simulink model "MPC_Speed_Control"  (R2024b)
settings: Solver=VariableStepAuto  StartTime=0.0  StopTime=50  RelTol=1e-3
model workspace (MAT data in the model file):
  I_max = Simulink.Parameter
  I_max.Complexity = 'real'
  I_max.Dimensions = [0 0]
  I_max.DataType = 'auto'
  Iq_max = Simulink.Parameter
  Iq_max.Value = 20
  Iq_max.Complexity = 'real'
  Iq_max.Dimensions = [1 1]
  Iq_max.DataType = 'double'
  Iq_max.Min = 0
  Iq_max.Max = 20
  Iq_max.DocUnits = 'A'
  Mech_Load = Simulink.Parameter
  Mech_Load.Value = 1
  Mech_Load.Complexity = 'real'
  Mech_Load.Dimensions = [1 1]
  Mech_Load.DataType = 'double'
  Mech_Load.Min = 0
  Mech_Load.Max = 20
libraries: spsCurrentMeasurementLib x3, spsSeriesRLCBranchLib x3, spsVoltageMeasurementLib x2, spsDCVoltageSourceLib x1, spsGroundLib x1, spsPermanentMagnetSynchronousMachineLib x1, spsUniversalBridgeLib x1, spsRMSLib x1, eeTransforms x1, slpidlib x1, spspowerguiLib x1
settings Model: ParameterArgumentNames=Iq_max,Mech_Load  Creator=hp  LastModifiedBy=hp
settings RTWCC: RTWVerbose=off

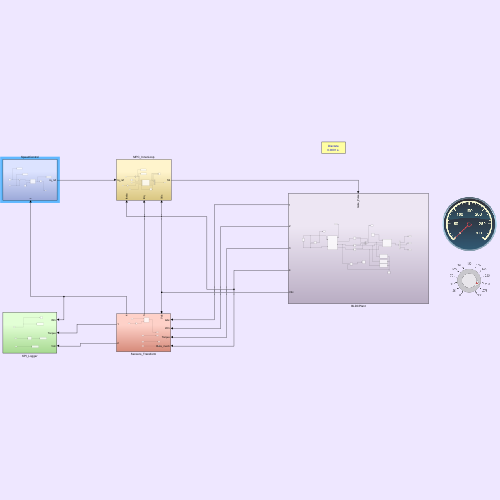
[thumbnail: Simulink's stored preview of the top-level diagram]
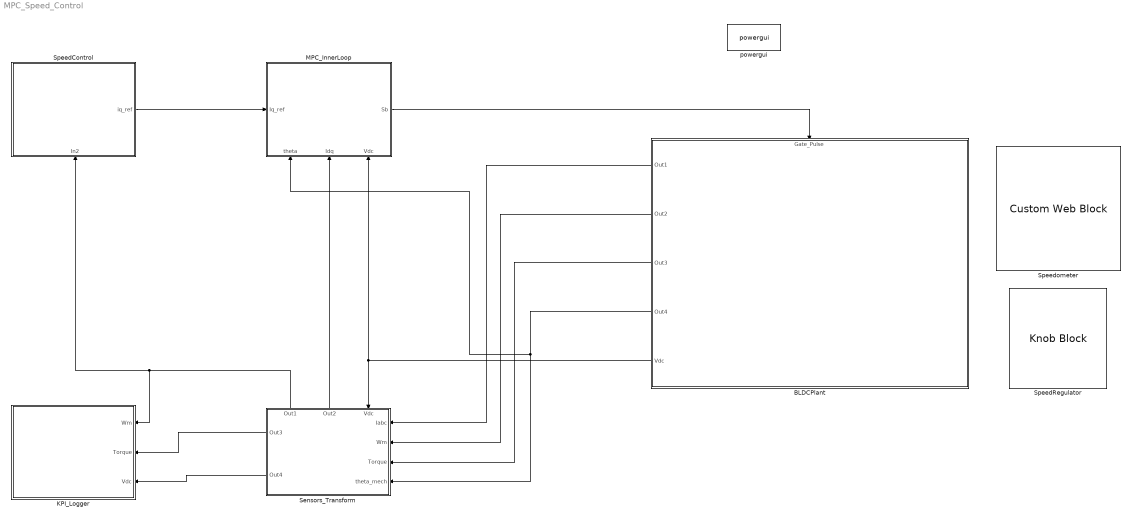
== system MPC_Speed_Control ==
  BLDCPlant : Subsystem
      settings: PortSchema="{\"entries\":[{\"content\":{\"sides\":[{\"content\":{},\"type\":\"ConnectorPlacement.EquallySpacedRectSide\",\"uuid\":\"b62d1c6e-a59d-4f65-8814-3dc177b23cd5\"},{\"content\":{\"connectorIds\":[\"Out1\",\"Out2\",\"Out3\",\"Out4\",\"Out5\"],\"side\":\"RIGHT\"},\"type\":\"ConnectorPlacement.EquallySpacedRectSide\",\"uuid\":\"6a33075d-b69e-43e0-847d-75198eb85e92\"},{\"content\":{\"connectorIds\":[\"In1\"],\"side\":\"TOP\"},\"type\":\"ConnectorPlacement.EquallySpacedRectSide\",\"uuid\":\"25902762-9f38-46cd-ae2e-4756f044da85\"}]},\"type\":\"ConnectorPlacement.EquallySpacedConnector\",\"uuid\":\"f42ce1bc-9199-4fe0-a1c0-02ea16a986e3\"}],\"packageUris\":[\"http://schema.mathworks.com/mf0/Connector/R2020b\"],\"version\":\"1.0\"}"
  KPI_Logger : Subsystem
  MPC_InnerLoop : Subsystem
      settings: PortSchema="{\"entries\":[{\"content\":{\"sides\":[{\"content\":{\"connectorIds\":[\"In1\"]},\"type\":\"ConnectorPlacement.EquallySpacedRectSide\",\"uuid\":\"1cededfe-a157-4693-a5d6-3ded835fc0fc\"},{\"content\":{\"connectorIds\":[\"Out1\"],\"side\":\"RIGHT\"},\"type\":\"ConnectorPlacement.EquallySpacedRectSide\",\"uuid\":\"33a5264e-419d-490c-8c5a-eb4ad8051faa\"},{\"content\":{\"side\":\"TOP\"},\"type\":\"ConnectorPlacement.EquallySpacedRectSide\",\"uuid\":\"1a0bf29c-4856-430c-b6c2-7eb59e496e99\"},{\"content\":{\"connectorIds\":[\"In2\",\"In3\",\"In4\"],\"side\":\"BOTTOM\"},\"type\":\"ConnectorPlacement.EquallySpacedRectSide\",\"uuid\":\"91ee846a-69f5-4705-a04e-f801c9f974eb\"}]},\"type\":\"ConnectorPlacement.EquallySpacedConnector\",\"uuid\":\"2fb1adc4-a0ec-4398-a1b1-d31f9fed8fac\"}],\"packageUris\":[\"http://schema.mathworks.com/mf0/Connector/R2020b\"],\"version\":\"1.0\"}"
  Sensors_Transform : Subsystem
      settings: PortSchema="{\"entries\":[{\"content\":{\"sides\":[{\"content\":{\"connectorIds\":[\"In1\",\"In2\",\"In3\",\"In4\"]},\"type\":\"ConnectorPlacement.EquallySpacedRectSide\",\"uuid\":\"6e3abafc-9605-4c64-93b2-a4bb92d8b15c\"},{\"content\":{\"connectorIds\":[\"Out1\",\"Out2\"],\"side\":\"RIGHT\"},\"type\":\"ConnectorPlacement.EquallySpacedRectSide\",\"uuid\":\"b2aa59f5-86cc-4d40-acb7-825075212f50\"},{\"content\":{\"connectorIds\":[\"In5\",\"Out3\",\"Out4\"],\"side\":\"TOP\"},\"type\":\"ConnectorPlacement.EquallySpacedRectSide\",\"uuid\":\"761892ed-2e7f-4fbb-8f28-8445ea92004b\"},{\"content\":{\"side\":\"BOTTOM\"},\"type\":\"ConnectorPlacement.EquallySpacedRectSide\",\"uuid\":\"9c48b8cc-eb13-4556-8d10-7bc854d50a3a\"}]},\"type\":\"ConnectorPlacement.EquallySpacedConnector\",\"uuid\":\"5da58205-14da-4f32-a3a9-21dbad898aea\"}],\"packageUris\":[\"http://schema.mathworks.com/mf0/Connector/R2020b\"],\"version\":\"1.0\"}"
  SpeedControl : Subsystem
      settings: PortSchema="{\"entries\":[{\"content\":{\"sides\":[{\"content\":{},\"type\":\"ConnectorPlacement.EquallySpacedRectSide\",\"uuid\":\"1cededfe-a157-4693-a5d6-3ded835fc0fc\"},{\"content\":{\"connectorIds\":[\"Out1\"],\"side\":\"RIGHT\"},\"type\":\"ConnectorPlacement.EquallySpacedRectSide\",\"uuid\":\"33a5264e-419d-490c-8c5a-eb4ad8051faa\"},{\"content\":{\"side\":\"TOP\"},\"type\":\"ConnectorPlacement.EquallySpacedRectSide\",\"uuid\":\"1a0bf29c-4856-430c-b6c2-7eb59e496e99\"},{\"content\":{\"connectorIds\":[\"In1\"],\"side\":\"BOTTOM\"},\"type\":\"ConnectorPlacement.EquallySpacedRectSide\",\"uuid\":\"33f77dac-6bdc-4222-b29b-be44d81ff2fe\"}]},\"type\":\"ConnectorPlacement.EquallySpacedConnector\",\"uuid\":\"2fb1adc4-a0ec-4398-a1b1-d31f9fed8fac\"}],\"packageUris\":[\"http://schema.mathworks.com/mf0/Connector/R2020b\"],\"version\":\"1.0\"}"
  SpeedRegulator : KnobBlock  LabelPosition=Hide  ScaleMax=300
  Speedometer : CustomWebBlock  LabelPosition=Hide  ShowInitialText=on  Configuration="{\"components\":[{\"name\":\"CircularScaleComponent\",\"settings\":{\"bounds\":{\"max\":300,\"min\":0,\"tickInterval\":\"auto\"},\"direction\":\"cw\",\"flipLimits\":0,\"innerRadius\":0.75,\"internalTickHeightScaleFactor\":1,\"labelColor\":[255,255,200],\"labelFont\":{\"font\":\"Arial\",\"fontSize\":12},\"labelRadius\":0.528,\"labelTransparency\":1,\"minorTickHeightScaleFactor\":0.2,\"needleImage\":{\"size\":[200,50],\"src\":\"data:image\\/svg+xml;base64,PD94bWwgdmVyc2lvbj0iMS4wIiBlbmNvZGluZz0idXRmLTgiPz4KPCEtLSBHZW5lcmF0b3I6IEFkb2JlIElsbHVzdHJhdG9yIDI0LjEuMiwgU1ZHIEV4cG9ydCBQbHVnLUluIC4gU1ZHIFZlcnNpb246IDYuMDAgQnVpbGQgMCkgIC0tPgo8c3ZnIHZlcnNpb249IjEuMSIgaWQ9IkxheWVyXzEiIHhtbG5zPSJodHRwOi8vd3d3LnczLm9yZy8yMDAwL3N2ZyIgeG1sbnM6eGxpbms9Imh0dHA6Ly93d3cudzMub3JnLzE5OTkveGxpbmsiIHg9IjBweCIgeT0iMHB4IgoJIHZpZXdCb3g9IjAgMCAyMDAgNTAiIHN0eWxlPSJlbmFibGUtYmFja2dyb3VuZDpuZXcgMCAwIDIwMCA1MDsiIHhtbDpzcGFjZT0icHJlc2VydmUiPgo8c3R5bGUgdHlwZT0idGV4dC9jc3MiPgoJLnN0MHtmaWxsOiNFQzIxMjc7fQo8L3N0eWxlPgo8cGF0aCBjbGFzcz0ic3QwIiBkPSJNMTYyLjgsMTMuN0MxNjksNC40LDE4MS43LDEuOSwxOTEsOC4xczExLjgsMTguOSw1LjYsMjguMnMtMTguOSwxMS44LTI4LjIsNS42bDAsMAoJQzE1OS4xLDM1LjYsMTU2LjYsMjMsMTYyLjgsMTMuN0wxNjIuOCwxMy43eiBNMTY1LjgsMTUuOGMtNS4xLDcuNi0zLjEsMTcuOSw0LjYsMjNjNy42LDUuMSwxNy45LDMuMSwyMy00LjYKCWM1LjEtNy42LDMuMS0xNy45LTQuNi0yM2wwLDBDMTgxLjIsNi4yLDE3MC45LDguMiwxNjUuOCwxNS44eiIvPgo8cGF0aCBjbGFzcz0ic3QwIiBkPSJNMC40LDI1Ljl2LTMuM2wxNTktMi41Yy0wLjcsMi42LTAuNyw1LjIsMCw3LjhMMC40LDI1Ljl6Ii8+CjxjaXJjbGUgY2xhc3M9InN0MCIgY3g9IjE3OS42IiBjeT0iMjQiIHI9IjAuNyIvPgo8L3N2Zz4K\"},\"needleOffset\":[0.18464878250906522,0],\"needleOrientation\":-45,\"needleRotation\":180,\"needleSize\":{\"height\":0.11741692305346914,\"width\":0.46108337545091255},\"outerRadius\":0.9,\"position\":[0.05,0.05,0.9,0.9],\"referencePoint\":\"auto\",\"scaleAngle\":270,\"scaleAngleOffset\":135,\"scaleColors\":[],\"scaleColorsSize\":0.2,\"scaleDirection\":\"CW\",\"scalePosition\":[0,0,1,1],\"showLabels\":1,\"showMinorTicks\":1,\"showSpanLine\":1,\"showTicks\":1,\"tickColor\":[252,252,197],\"tickTransparency\":1,\"valueBarColor\":[0,114,189],\"valueBarPosition\":[0,0,1,1],\"valueBarSize\":0.2,\"valueBarTransparency\":1}},{\"name\":\"BackgroundImageComponent\",\"settings\":{\"image\":{\"size\":[500,500],\"src\":\"data:image\\/svg+xml;base64,PD94bWwgdmVyc2lvbj0iMS4wIiBlbmNvZGluZz0iVVRGLTgiIHN0YW5kYWxvbmU9Im5vIj8+CjxzdmcKICAgeG1sbnM6ZGM9Imh0dHA6Ly9wdXJsLm9yZy9kYy9lbGVtZW50cy8xLjEvIgogICB4bWxuczpjYz0iaHR0cDovL2NyZWF0aXZlY29tbW9ucy5vcmcvbnMjIgogICB4bWxuczpyZGY9Imh0dHA6Ly93d3cudzMub3JnLzE5OTkvMDIvMjItcmRmLXN5bnRheC1ucyMiCiAgIHhtbG5zOnN2Zz0iaHR0cDovL3d3dy53My5vcmcvMjAwMC9zdmciCiAgIHhtbG5zPSJodHRwOi8vd3d3LnczLm9yZy8yMDAwL3N2ZyIKICAgeG1sbnM6 ...(+9964 chars)\"},\"position\":[0,0,1,1],\"scaleMode\":\"0\"}},{\"name\":\"ForegroundImageComponent\",\"settings\":{\"image\":{\"size\":[0,0],\"src\":\"default\",\"srcOrientation\":[]},\"isForeground\":1,\"position\":[0,0,1,1],\"scaleMode\":\"0\"}}],\"settings\":{\"BindingType\":\"signal\",\"aspectRatio\":1.032258064516129,\"backgroundColor\":[0,0,0,\"1\"],\"backgroundOffset\":1,\"backgroundOpacity\":1,\"direction\":\"cw\",\"fixedAspectRatio\":\"on\",\"flipLimits\":0,\"orientation\":\"horizontal\",\"showBackgroundColor\":false,\"value\":0,\"version\":\"R2023a\"},\"type\":\"CircularGauge\"}"
  powergui : spspowerguiLib/powergui  Priority=1  SimulationMode=Discrete  SampleTime=100*1e-6  frequency=60  Iterations=50  frequencyindice=0  Pbase=100e6  ErrMax=1e-4  UnitsV=kV  UnitsW=MW  buscounter=0  FunctionMessages=off  echomessages=off  EnableUseOfTLC=off  CurrentSourceSwitches=off  DisableSnubberDevices=off  DisableRonSwitches=off  DisableVfSwitches=off  DisplayEquations=off  AutomaticDiscreteSolvers=off  SolverType=Tustin/Backward Euler (TBE)  Interpol=off  ExternalGateDelay=off  methode=off  Ts=100  x0status=blocks  SPID=on  SwTol=0  HookPort=off  NonlinearTolerance=1e-4  nMaxIteration=100  ContinueOnMaxIteration=off  RestoreLinks=warning  ResistiveCurrentMeasurement=off  Frange=[0:2:500]  Ylog=off  Xlog=on  ShowGrid=off  save=off  variable=ZData  structure=0  ZoomFFT=off  StartTime=0.0  cycles=1  DisplayStyle=1  fundamental=60  FreqAxis=off  MaxFrequency=1000  frequencyindicesteady=1  RmsSteady=1  display=off
  wires:
  SpeedControl/1(iq_ref) -> MPC_InnerLoop/1(Iq_ref)
  MPC_InnerLoop/1(Sb) -> BLDCPlant/1(Gate_Pulse)
  BLDCPlant/1(Out1) -> Sensors_Transform/1(Iabc)
  Sensors_Transform/4(Out1) -> SpeedControl/1(In2), KPI_Logger/1(Wm)
  Sensors_Transform/3(Out2) -> MPC_InnerLoop/3(Idq)
  Sensors_Transform/1(Out3) -> KPI_Logger/2(Torque)
  BLDCPlant/3(Out3) -> Sensors_Transform/3(Torque)
  BLDCPlant/4(Out4) -> MPC_InnerLoop/2(theta), Sensors_Transform/4(theta_mech)
  BLDCPlant/2(Out2) -> Sensors_Transform/2(Wm)
  BLDCPlant/5(Vdc) -> Sensors_Transform/5(Vdc), MPC_InnerLoop/4(Vdc)
  Sensors_Transform/2(Out4) -> KPI_Logger/3(Vdc)

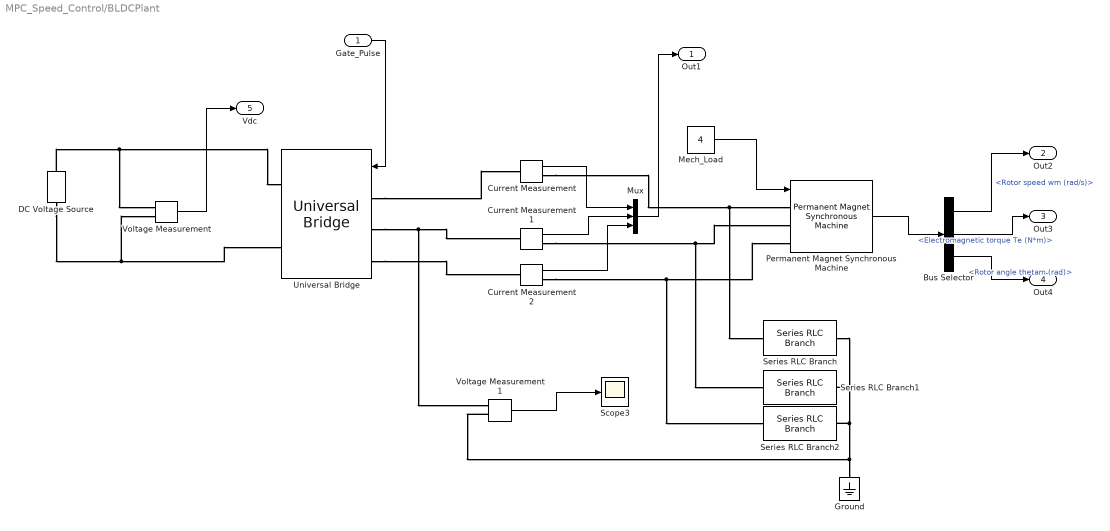
== system MPC_Speed_Control/BLDCPlant ==
  Gate_Pulse : Inport
  Bus Selector : BusSelector  OutputSignals=Rotor speed wm (rad/s),Electromagnetic torque Te (N*m),Rotor angle thetam (rad)
  Current Measurement : spsCurrentMeasurementLib/Current Measurement  PhasorSimulation=off  OutputType=Complex  PSBequivalent=0
  Current Measurement1 : spsCurrentMeasurementLib/Current Measurement  PhasorSimulation=off  OutputType=Complex  PSBequivalent=0
  Current Measurement2 : spsCurrentMeasurementLib/Current Measurement  PhasorSimulation=off  OutputType=Complex  PSBequivalent=0
  DC Voltage Source : spsDCVoltageSourceLib/DC Voltage Source  Amplitude=400  Measurements=None
  Ground : spsGroundLib/Ground  LConnTagsString=a
  Mech_Load : Constant  Value=4  SampleTime=-1
  Mux : Mux  Inputs=3
  Permanent Magnet Synchronous Machine : spsPermanentMagnetSynchronousMachineLib/Permanent Magnet Synchronous Machine  NbPhases=3  FluxDistribution=Trapezoidal  RotorType=Round  MechanicalLoad=Torque Tm  PresetModel=No  ShowDetailedParameters=on  MeasurementBus=off  Resistance=0.0485  Inductance=8.5e-3  dqInductances=[8.5e-3,8.5e-3]  La=0.000395  MachineConstant=Flux linkage established by magnets (V.s)  Flux=0.1194  VoltageCst=50.0142  TorqueCst=0.4776  Flat=120  Mechanical=[0.0027 0.0004924 2 0]  PolePairs=4  InitialConditions=[0,0, 0,0]  InitialConditions5ph=[0 0 0 0 0 0]  RefAngle=Aligned with phase A axis (original Park)  IterativeDiscreteModel=Trapezoidal robust  TsBlock=-1  TsPowergui=0
  Scope3 : Scope
  Series RLC Branch : spsSeriesRLCBranchLib/Series RLC Branch  LConnTagsString=__new0  RConnTagsString=__new0  BranchType=R  Resistance=100  Inductance=1e-3  SetiL0=off  InitialCurrent=0  Capacitance=1e-6  Setx0=off  InitialVoltage=0  Measurements=None
  Series RLC Branch1 : spsSeriesRLCBranchLib/Series RLC Branch  LConnTagsString=__new0  RConnTagsString=__new0  BranchType=R  Resistance=100  Inductance=1e-3  SetiL0=off  InitialCurrent=0  Capacitance=1e-6  Setx0=off  InitialVoltage=0  Measurements=None
  Series RLC Branch2 : spsSeriesRLCBranchLib/Series RLC Branch  LConnTagsString=__new0  RConnTagsString=__new0  BranchType=R  Resistance=100  Inductance=1e-3  SetiL0=off  InitialCurrent=0  Capacitance=1e-6  Setx0=off  InitialVoltage=0  Measurements=None
  Universal Bridge : spsUniversalBridgeLib/Universal Bridge  Arms=3  SnubberResistance=100  SnubberCapacitance=1e-7  Device=IGBT / Diodes  Ron=1e-3  Lon=0  ForwardVoltages="[  0  0  ]"  ForwardVoltage=0  GTOparameters=[ 10e-6 , 20e-6 ]  IGBTparameters=[ 1e-6 , 2e-6 ]  Measurements=None  Measurements_2=None  converterType=Rectifier
  Voltage Measurement : spsVoltageMeasurementLib/Voltage Measurement  PhasorSimulation=off  OutputType=Complex  PSBequivalent=0
  Voltage Measurement1 : spsVoltageMeasurementLib/Voltage Measurement  PhasorSimulation=off  OutputType=Complex  PSBequivalent=0
  Out1 : Outport
  Out2 : Outport  Port=2
  Out3 : Outport  Port=3
  Out4 : Outport  Port=4
  Vdc : Outport  Port=5
  wires:
  Mux/1 -> Out1/1
  Mech_Load/1 -> Permanent Magnet Synchronous Machine/1
  Voltage Measurement/1 -> Vdc/1
  Current Measurement/1 -> Mux/1
  Current Measurement1/1 -> Mux/2
  Current Measurement2/1 -> Mux/3
  Permanent Magnet Synchronous Machine/1 -> Bus Selector/1
  Gate_Pulse/1 -> Universal Bridge/1
  Voltage Measurement1/1 -> Scope3/1
  Bus Selector/3 -> Out4/1  "<Rotor angle thetam (rad)>"
  Bus Selector/2 -> Out3/1  "<Electromagnetic torque Te (N*m)>"
  Bus Selector/1 -> Out2/1  "<Rotor speed wm (rad/s)>"
  connections:
  Universal Bridge/LConn1 -- Current Measurement/LConn1
  Universal Bridge/LConn2 -- Voltage Measurement1/LConn1 -- Current Measurement1/LConn1
  Universal Bridge/LConn3 -- Current Measurement2/LConn1
  Current Measurement/RConn1 -- Series RLC Branch/LConn1 -- Permanent Magnet Synchronous Machine/LConn1
  Current Measurement1/RConn1 -- Series RLC Branch1/LConn1 -- Permanent Magnet Synchronous Machine/LConn2
  Current Measurement2/RConn1 -- Series RLC Branch2/LConn1 -- Permanent Magnet Synchronous Machine/LConn3
  DC Voltage Source/RConn1 -- Voltage Measurement/LConn1 -- Universal Bridge/RConn1
  DC Voltage Source/LConn1 -- Universal Bridge/RConn2 -- Voltage Measurement/LConn2
  Series RLC Branch/RConn1 -- Voltage Measurement1/LConn2 -- Ground/LConn1 -- Series RLC Branch2/RConn1 -- Series RLC Branch1/RConn1

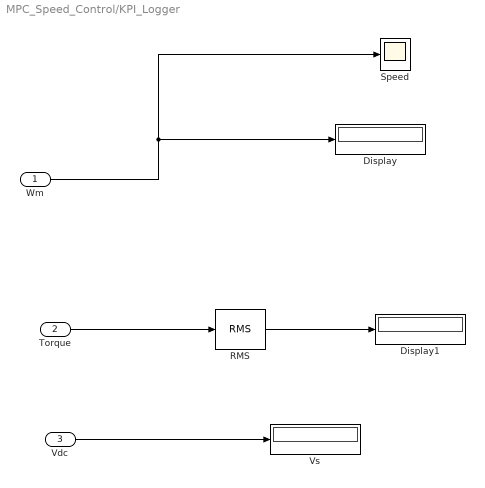
== system MPC_Speed_Control/KPI_Logger ==
  Wm : Inport
  Torque : Inport  Port=2
  Vdc : Inport  Port=3
  Display : Display
  Display1 : Display
  RMS : spsRMSLib/RMS  TrueRMS=on  Freq=60  RMSInit=120  Ts=0
  Speed : Scope
  Vs : Display
  wires:
  Wm/1 -> Speed/1, Display/1
  Vdc/1 -> Vs/1
  Torque/1 -> RMS/1
  RMS/1 -> Display1/1

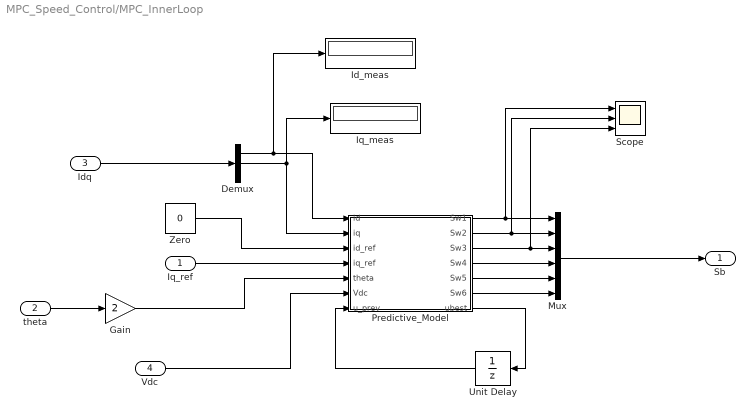
== system MPC_Speed_Control/MPC_InnerLoop ==
  Iq_ref : Inport
  theta : Inport  Port=2
  Idq : Inport  Port=3
  Vdc : Inport  Port=4
  Demux : Demux  Outputs=3
  Gain : Gain  Gain=2
  Id_meas : Display
  Iq_meas : Display
  Mux : Mux  Inputs=6
  Predictive_Model : MATLAB Function  TreatAsAtomicUnit=on  SystemSampleTime=100*1e-6
  Scope : Scope  NumInputPorts=3
  Unit Delay : UnitDelay  SampleTime=-1  HasFrameUpgradeWarning=on
  Zero : Constant  Value=0  OutDataTypeStr=Inherit: Inherit via back propagation  SampleTime=-1
  Sb : Outport
  wires:
  Demux/1 -> Id_meas/1, Predictive_Model/1(id)
  theta/1 -> Gain/1
  Idq/1 -> Demux/1
  Vdc/1 -> Predictive_Model/6(Vdc)
  Gain/1 -> Predictive_Model/5(theta)
  Iq_ref/1 -> Predictive_Model/4(iq_ref)
  Demux/2 -> Predictive_Model/2(iq), Iq_meas/1
  Predictive_Model/7(ubest) -> Unit Delay/1
  Zero/1 -> Predictive_Model/3(id_ref)
  Unit Delay/1 -> Predictive_Model/7(u_prev)
  Predictive_Model/1(Sw1) -> Scope/1, Mux/1
  Predictive_Model/2(Sw2) -> Scope/2, Mux/2
  Predictive_Model/3(Sw3) -> Scope/3, Mux/3
  Predictive_Model/4(Sw4) -> Mux/4
  Predictive_Model/5(Sw5) -> Mux/5
  Predictive_Model/6(Sw6) -> Mux/6
  Mux/1 -> Sb/1

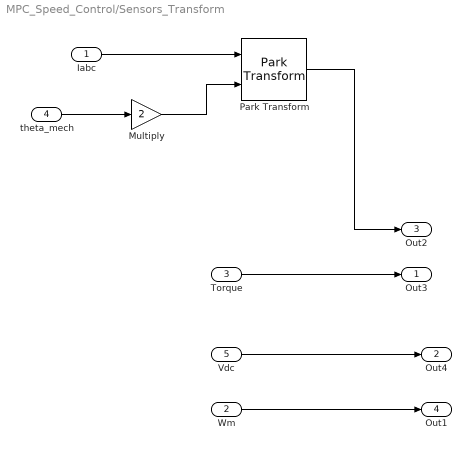
== system MPC_Speed_Control/Sensors_Transform ==
  Iabc : Inport  SampleTime=100*1e-6
  Wm : Inport  Port=2
  Torque : Inport  Port=3
  theta_mech : Inport  Port=4  SampleTime=100*1e-6
  Vdc : Inport  Port=5
  Multiply : Gain  Gain=2
  Park Transform : eeTransforms/Park Transform  AxisAlignment=D-axis  PowerInvariant=off
      settings: LibrarySourceBlock=|
      | ee_sl_lib/Mathematical
      | Transforms/Park Transform
  Out3 : Outport
  Out4 : Outport  Port=2
  Out2 : Outport  Port=3
  Out1 : Outport  Port=4
  wires:
  Iabc/1 -> Park Transform/1
  theta_mech/1 -> Multiply/1
  Multiply/1 -> Park Transform/2
  Park Transform/1 -> Out2/1
  Wm/1 -> Out1/1
  Torque/1 -> Out3/1
  Vdc/1 -> Out4/1

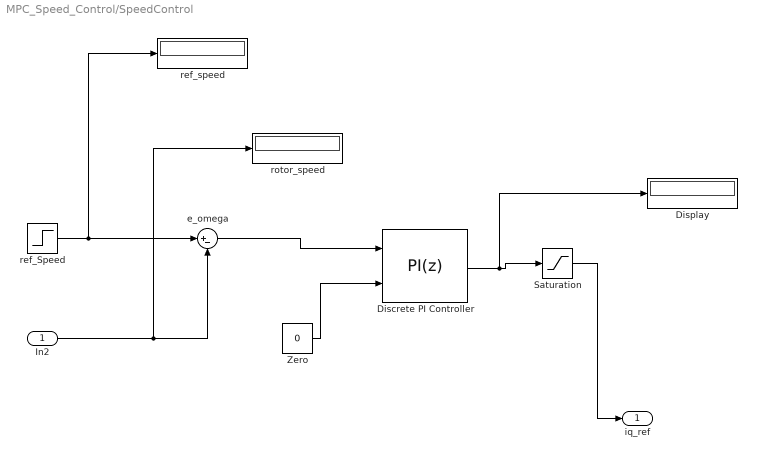
== system MPC_Speed_Control/SpeedControl ==
  In2 : Inport
  Discrete PI Controller : slpidlib/PID Controller  Controller=PI  Form=Parallel  TimeDomain=Discrete-time  UseExternalTs=off  SampleTime=0.001  IntegratorMethod=Forward Euler  FilterMethod=Forward Euler  ControllerParametersSource=internal  P=0.1  I=3  UseKiTs=off  D=0  UseExternalDerivativeSource=off  N=100  UseFilter=on  TunerSelectOption=Transfer Function Based (PID Tuner App)  InitialConditionSource=external  InitialConditionForIntegrator=0  InitialConditionForFilter=0  DifferentiatorICPrevScaledInput=0  ExternalReset=none  TrackingMode=off  Kt=1  LimitOutput=on  SatLimitsSource=internal  UpperSaturationLimit=20  LowerSaturationLimit=0  LinearizeAsGain=off  AntiWindupMode=back-calculation  Kb=1  LimitIntegrator=off  UpperIntegratorSaturationLimit=inf  LowerIntegratorSaturationLimit=-inf  POutMin=[]  POutMax=[]  IOutMin=[]  IOutMax=[]  DOutMin=[]  DOutMax=[]  NOutMin=[]  NOutMax=[]  SumOutMin=[]  SumOutMax=[]  SaturationOutMin=[]  SaturationOutMax=[]  PParamMin=[]  PParamMax=[]  IParamMin=[]  IParamMax=[]  DParamMin=[]  DParamMax=[]  NParamMin=[]  NParamMax=[]  KbParamMin=[]  KbParamMax=[]  KtParamMin=[]  KtParamMax=[]  KbOutMin=[]  KbOutMax=[]  KtOutMin=[]  KtOutMax=[]  IntegratorOutMin=[]  IntegratorOutMax=[]  FilterOutMin=[]  FilterOutMax=[]  SumI1OutMin=[]  SumI1OutMax=[]  SumI2OutMin=[]  SumI2OutMax=[]  SumI3OutMin=[]  SumI3OutMax=[]  SumI4OutMin=[]  SumI4OutMax=[]  SumDOutMin=[]  SumDOutMax=[]  DifferentiatorOutMin=[]  DifferentiatorOutMax=[]  FilterDiffOutCoefMin=[]  FilterDiffOutCoefMax=[]  ReciprocalOutMin=[]  ReciprocalOutMax=[]  SumDenOutMin=[]  SumDenOutMax=[]  SumNumOutMin=[]  SumNumOutMax=[]  DivideOutMin=[]  DivideOutMax=[]  UdiffTsProdOutMin=[]  UdiffTsProdOutMax=[]  NTsProdOutMin=[]  NTsProdOutMax=[]  UintegralTsProdOutMin=[]  UintegralTsProdOutMax=[]  UngainTsProdOutMin=[]  UngainTsProdOutMax=[]  ClampingZeroOutDataTypeStr=Inherit: Inherit via back propagation  ClampingZeroOutMin=[]  ClampingZeroOutMax=[]  FilterDenConstantOutDataTypeStr=Inherit: Inherit via back propagation  FilterDenConstantOutMin=[]  FilterDenConstantOutMax=[]  PCopyOutDataTypeStr=Inherit: Inherit via back propagation  PCopyOutMin=[]  PCopyOutMax=[]  NCopyOutDataTypeStr=Inherit: Inherit via back propagation  NCopyOutMin=[]  NCopyOutMax=[]  IntegratorContinuousStateAttributes=''  IntegratorStateMustResolveToSignalObject=off  IntegratorRTWStateStorageClass=Auto  FilterContinuousStateAttributes=''  FilterStateMustResolveToSignalObject=off  FilterRTWStateStorageClass=Auto  ParallelPVariant=InternalParameters  IdealPVariant=Disabled  IVariant=InternalParameters  DVariant=Disabled  IntegratorVariant=Discrete  SatVariant=Enabled  AWVariant=BackCalculation  PCopyVariant=Disabled  TRVariant=Disabled  FdbkBlocksVariant=Forward  IdealPFdbkVariant=Disabled  SatFdbkVariant=Disabled  DerivativeFilterVariant=Disabled  NVariant=Disabled  NCopyVariant=Disabled_SignalSpec  FilterICVariant=Disabled  IntegratorICVariant=ExternalICs  ExternalResetVariant=Disabled  TRSumVariant=Passthrough  SumFdbkVariant=Disabled  SumVariant=Sum_PI  TsampFilterVariant=InternalTs  TsampNgainVariant=Passthrough  TsampIntegralVariant=Disabled_SignalSpec  ExternalSaturationOutDataTypeStr=Inherit: Same as second input  DerivativeSourceVariant=Disabled  PreIntVariant=InternalPreInt
      settings: LibrarySourceBlock=simulink/Discrete/Discrete PID Controller
  Display : Display
  Saturation : Saturate  UpperLimit=Iq_max  LowerLimit=0
  Zero : Constant  Value=0  OutDataTypeStr=Inherit: Inherit via back propagation
  e_omega : Sum  Inputs=|+-
  ref_Speed : Step  After=258.916983034877  SampleTime=0.001
  ref_speed : Display
  rotor_speed : Display
  iq_ref : Outport
  wires:
  Zero/1 -> Discrete PI Controller/2
  e_omega/1 -> Discrete PI Controller/1
  Discrete PI Controller/1 -> Display/1, Saturation/1
  Saturation/1 -> iq_ref/1
  In2/1 -> rotor_speed/1, e_omega/2
  ref_Speed/1 -> ref_speed/1, e_omega/1

== matlab function MPC_Speed_Control/MPC_InnerLoop/Predictive_Model ==
  data: id input; Sw1 output; Sw2 output; Sw3 output; Sw4 output; Sw5 output; Sw6 output; iq input; id_ref input; iq_ref input; theta input; Vdc input; u_prev input; ubest output
function [Sw1,Sw2,Sw3,Sw4,Sw5,Sw6,ubest] = fcsmpc_dq(id, iq, id_ref, iq_ref, theta, Vdc, u_prev)
%#codegen
% Inputs:  id, iq (A), id_ref, iq_ref, electrical theta (rad), Vdc (V), u_prev in {0..7}
% Outputs: Sa,Sb,Sc as logical gate states; ubest in {0..7}

% ---- Motor / control params ----
Rs   = 0.35;
Ld   = 0.00025;
Lq   = 0.00025;
lam_f= 0.035;
p    = 4;          %#ok<NASGU>  % not used here but kept for clarity
Ts   = 20e-6;      % MUST match your controller sample time
alpha_i  = 1.0;
alpha_sw = 0.02;
Imax = 20;

% 8 inverter states (Sa Sb Sc)
S =      ([0 0 0;
           1 0 0;
           1 1 0;
           0 1 0;
           0 1 1;
           0 0 1;
           1 0 1;
           1 1 1]);

% ---- persistent for speed estimate ----
persistent theta_prev
if isempty(theta_prev)
    theta_prev = theta;
end
dtheta  = theta - theta_prev;
% wrap to [-pi, pi] to avoid spikes across 2π
dtheta  = atan2(sin(dtheta), cos(dtheta));
omega_e = dtheta / Ts;
theta_prev = theta;

% ---- initialize outputs with fixed size & type ----
Sw1 = false;
Sw2 = false;
Sw3 = false;
Sw4 = false;
Sw5 = false;
Sw6 = false;     % logical

ubest = double(0);  % {0..7}

Jbest = inf;

% ---- precompute trig ----
c = cos(theta);
s = sin(theta);

% ---- loop candidates ----
for ui =1:8
    Sa_c = double(S(ui,1));
    Sb_c = double(S(ui,2));
    Sc_c = double(S(ui,3));

    % Two-level inverter αβ voltages (line-neutral), normalized
    v_alpha = (2/3)*Vdc*( Sa_c - 0.5*Sb_c - 0.5*Sc_c );
    v_beta  = (2/3)*Vdc*( (sqrt(3)/2)*(Sb_c - Sc_c) );

    % αβ -> dq
    vd =  c*v_alpha + s*v_beta;
    vq = -s*v_alpha + c*v_beta;

    % one-step prediction (Euler)
    did = (vd - Rs*id + omega_e*Lq*iq) / Ld;
    diq = (vq - Rs*iq - omega_e*Ld*id - omega_e*lam_f) / Lq;
    id1 = id + Ts*did;
    iq1 = iq + Ts*diq;

    % soft clamp
    if id1 >  Imax, id1 =  Imax; end
    if id1 < -Imax, id1 = -Imax; end
    if iq1 >  Imax, iq1 =  Imax; end
    if iq1 < -Imax, iq1 = -Imax; end

    % cost
    Ji = alpha_i*((id1 - id_ref)^2 + (iq1 - iq_ref)^2) ...
       + alpha_sw*(double(ui) - double(u_prev))^2;

    % select best
    if Ji < Jbest
        Jbest = Ji;
        ubest = double(ui);                       % 1..8
        Sw1    = logical(S(ui,1));
        Sw3    = logical(S(ui,2));
        Sw5    = logical(S(ui,3));
        Sw2    = ~Sw5;
        Sw4    = ~Sw1;
        Sw6    = ~Sw3;

    end
end
end
